simulink model "PROYECTO_ING_CONTROL"  (R2021b)
settings: Solver=ode4  StartTime=0.0  StopTime=30  FixedStep=0.001  RelTol=1e-3
settings Model: Creator=mluser  LastModifiedBy=mluser

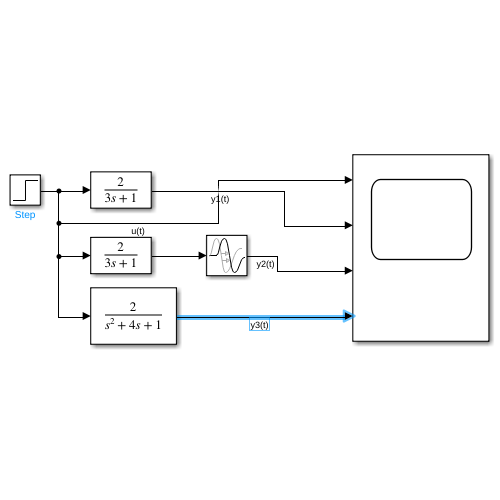
[thumbnail: Simulink's stored preview of the top-level diagram]
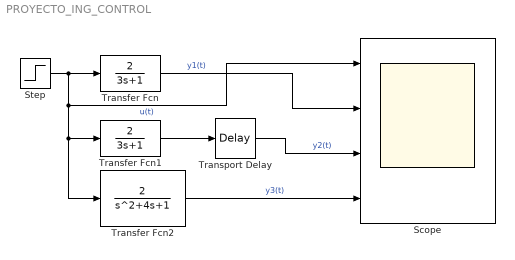
== system PROYECTO_ING_CONTROL ==
  Scope : Scope  NumInputPorts=4
  Step : Step  Time=0  After=10  SampleTime=0
  Transfer Fcn : TransferFcn  Numerator=[2]  Denominator=[3 1]
  Transfer Fcn1 : TransferFcn  Numerator=[2]  Denominator=[3 1]
  Transfer Fcn2 : TransferFcn  Numerator=[2]  Denominator=[1 4 1]
  Transport Delay : TransportDelay  DelayTime=4
  wires:
  Step/1 -> Scope/1, Transfer Fcn2/1, Transfer Fcn1/1, Transfer Fcn/1  "u(t)"
  Transfer Fcn/1 -> Scope/2  "y1(t)"
  Transfer Fcn1/1 -> Transport Delay/1
  Transport Delay/1 -> Scope/3  "y2(t)"
  Transfer Fcn2/1 -> Scope/4  "y3(t)"
